simulink model "autoMBD_example_PI_vSubs"  (R2020b)
settings: Solver=FixedStepAuto  StartTime=0.0  StopTime=10.0  FixedStep=0.001  RelTol=1e-3
undefined symbols (not defined in the file or in its folder): DiscIntNeverNeededParam
settings Model: Creator=k  LastModifiedBy=k
settings OptimizationCC: DefaultParameterBehavior=Inlined  EnhancedBackFolding=on  PassReuseOutputArgsAs=Individual arguments  ZeroExternalMemoryAtStartup=off  ZeroInternalMemoryAtStartup=off  OptimizeBlockOrder=speed  DifferentSizesBufferReuse=on  OptimizationCustomize=off  EfficientTunableParamExpr=on
settings DebuggingCC: ParameterTunabilityLossMsg=error
settings SFSimCC: MATLABDynamicMemAlloc=off
settings RTWCC: Description=Embedded Coder  SystemTargetFile=ert.tlc  GenCodeOnly=on  TemplateMakefile=ert_default_tmf
settings CodeAppCC: ForceParamTrailComments=on  IgnoreCustomStorageClasses=off  OperatorAnnotations=on  SimulinkDataObjDesc=on  SFDataObjDesc=on  InsertBlockDesc=on
settings ERTTargetCC: TargetLangStandard=C99 (ISO)  GenerateSampleERTMain=on  InlinedParameterPlacement=NonHierarchical  ERTCustomFileTemplate=example_file_process.tlc

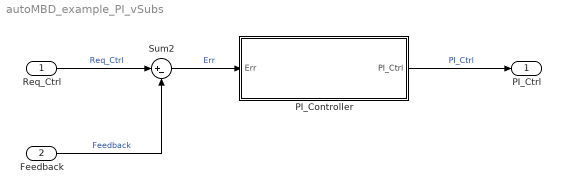
== system autoMBD_example_PI_vSubs ==
  Req_Ctrl : Inport
  Feedback : Inport  Port=2
  PI_Controller : Subsystem
  Sum2 : Sum  Inputs=|+-
  PI_Ctrl : Outport
  wires:
  Req_Ctrl/1 -> Sum2/1  "Req_Ctrl"
  Feedback/1 -> Sum2/2  "Feedback"
  Sum2/1 -> PI_Controller/1(Err)  "Err"
  PI_Controller/1(PI_Ctrl) -> PI_Ctrl/1  "PI_Ctrl"

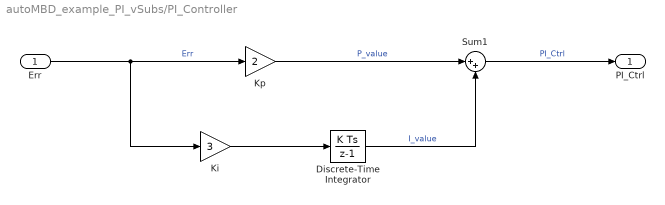
== system autoMBD_example_PI_vSubs/PI_Controller ==
  Err : Inport
  Discrete-Time Integrator : DiscreteIntegrator  SampleTime=-1  ICPrevOutput=DiscIntNeverNeededParam  ICPrevScaledInput=DiscIntNeverNeededParam
  Ki : Gain  Gain=3
  Kp : Gain  Gain=2
  Sum1 : Sum  Inputs=|++
  PI_Ctrl : Outport
  wires:
  Sum1/1 -> PI_Ctrl/1  "PI_Ctrl"
  Err/1 -> Ki/1, Kp/1  "Err"
  Discrete-Time Integrator/1 -> Sum1/2  "I_value"
  Ki/1 -> Discrete-Time Integrator/1
  Kp/1 -> Sum1/1  "P_value"
